simulink model "ProbeklausurLoesungR2021"  (R2021b)
settings: Solver=ode1  StartTime=0.0  StopTime=20  FixedStep=0.00001  RelTol=1e-3
values from neighbouring files (symbols this model uses):
  m = 4    [integrieren.m]
undefined symbols (not defined in the file or in its folder): C2
settings Model: Creator=PM  LastModifiedBy=metzler
settings SolverCC: AlgebraicLoopSolver=TrustRegion
settings DebuggingCC: AlgebraicLoopMsg=none  UnconnectedInputMsg=none  UnconnectedOutputMsg=none  UnconnectedLineMsg=none
settings ModelReferenceCC: EnableRefExpFcnMdlSchedulingChecks=off

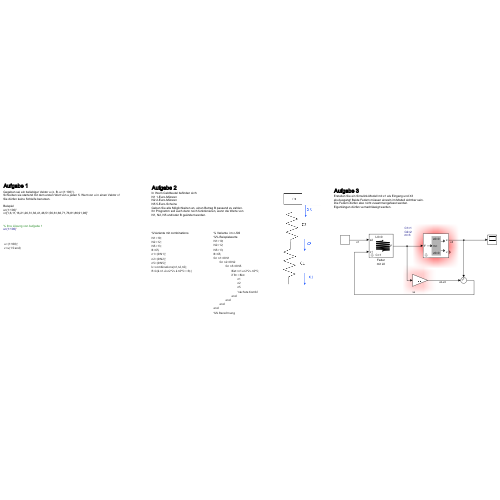
[thumbnail: Simulink's stored preview of the top-level diagram]
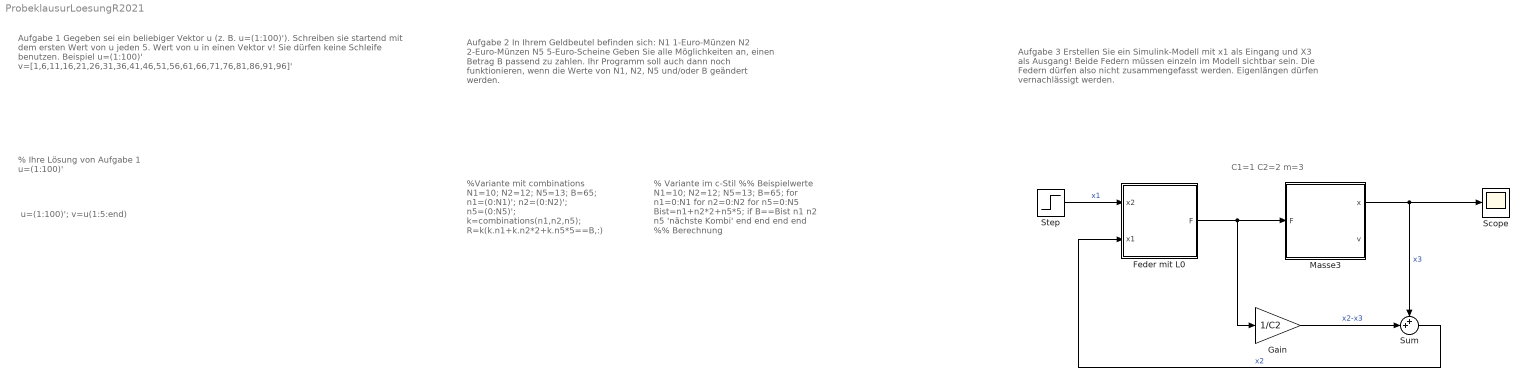
== system ProbeklausurLoesungR2021 ==
  note: Aufgabe 2
      | In Ihrem Geldbeutel befinden sich:
      | N1 1-Euro-Münzen
      | N2 2-Euro-Münzen
      | N5 5-Euro-Scheine
      | Geben Sie alle Möglichkeiten an, einen Betrag B passend zu zahlen.
      | Ihr Programm soll auch dann noch funktionieren, wenn die Werte von
      | N1, N2, N5 und/oder B geändert werden.
  note: Aufgabe 1
      | Gegeben sei ein beliebiger Vektor u (z. B. u=(1:100)').
      | Schreiben sie startend mit dem ersten Wert von u jeden 5. Wert von u in einen Vektor v!
      | Sie dürfen keine Schleife benutzen.
      |
      | Beispiel
      | u=(1:100)'
      | v=[1,6,11,16,21,26,31,36,41,46,51,56,61,66,71,76,81,86,91,96]'
  note: % Ihre Lösung von Aufgabe 1
      | u=(1:100)'
  note: Aufgabe 3
      | Erstellen Sie ein Simulink-Modell mit x1 als Eingang und X3
      | als Ausgang! Beide Federn müssen einzeln im Modell sichtbar sein.
      | Die Federn dürfen also nicht zusammengefasst werden.
      | Eigenlängen dürfen vernachlässigt werden.
  note: u=(1:100)';
      | v=u(1:5:end)
  note: %Variante mit combinations
      | N1=10;
      | N2=12;
      | N5=13;
      | B=65;
      | n1=(0:N1)';
      | n2=(0:N2)';
      | n5=(0:N5)';
      | k=combinations(n1,n2,n5);
      | R=k(k.n1+k.n2*2+k.n5*5==B,:)
  note: % Variante im c-Stil
      | %% Beispielwerte
      | N1=10;
      | N2=12;
      | N5=13;
      | B=65;
      | for n1=0:N1
      | for n2=0:N2
      | for n5=0:N5
      | Bist=n1+n2*2+n5*5;
      | if B==Bist
      | n1
      | n2
      | n5
      | 'nächste Kombi'
      | end
      | end
      | end
      | end
      | %% Berechnung
  note: C1=1
      | C2=2
      | m=3
  " Feder mit L0" : Subsystem  mask{C=1, L0=0}
      mask prompts: C "Spring Constant C [N/m]"; L0 "Length of Spring if no force is applied L0 [m]"
      mask help:
      | If no force F is applied, the spring has the length L0.
      |
      | F=C*sign(x2-x1-L0)*((x2-x1-L0)
      mask Display:
      | plot(20,0)
      | plot(90,100)
      | plot([60,60],[25,30])
      | plot([60,80],[30,32])
      | plot([80,40],[32,36])
      | plot([40,80],[36,40])
      | plot([80,40],[40,44])
      | plot([40,80],[44,48])
      | plot([80,40],[48,52])
      | plot([40,80],[52,56])
      | plot([80,40],[56,60])
      | plot([40,80],[60,64])
      | plot([80,40],[64,68])
      | plot([40,60],[68,70])
      | plot([60,60],[70,75])
      | 
      | 
      | port_label ('output',1,'F')
      | port_label ('input',1,'x2')
      | port_label ('input',2,'x1')
      | 
      | text(40,10,['C=',num2str(C)])
      | text(40,90,['L0=',num2str(L0)])
  Gain : Gain  Gain=1/C2
  Masse3 : Subsystem  mask{m=m, v0=0, x0=0}
      mask prompts: m "Masse m"; v0 "Anfangsgeschwindigkeit v_0"; x0 "Anfangsposition x_0"
      mask help:
      | Calculates the position s and the velocity v of a mass as a function of the Force F and the initial velocity v_0 and initial position s_0.
      | Berechnet die Position und die Geschwindigkeit eines Köpers mit der Masse m. Auf den Köper wirkt die Kraft F. Die Anfangsposition ist s_0, die Anfangsgeschwindigkeit ist v_0.
      mask Display:
      | plot(0,0)
      | plot(100,100)
      | patch([35 35 70 70],[10 90 90 10],[0.7,0.7,0.7])
      | text(40,80,['x0=',num2str(x0)])
      | text(40,50,['m=',num2str(m)])
      | text(40,20,['v0=',num2str(v0)])
      | plot([70 80],[70 70])
      | patch([80 80 85],[65 75 70],[0 0 0])
      | plot([15 35],[50 50])
      | patch([30 30 35],[45 55 50],[0 0 0])
      | plot([70 80],[30 30])
      | patch([80 80 85],[25 35 30],[0 0 0])
      | port_label ('output',1,'x')
      | port_label ('output',2,'v')
      | port_label ('input',1,'F')
  Scope : Scope
  Step : Step  SampleTime=0
  Sum : Sum  Inputs=++|
  wires:
  Sum/1 -> " Feder mit L0"/2(x1)  "x2"
  " Feder mit L0"/1(F) -> Gain/1, Masse3/1(F)
  Step/1 -> " Feder mit L0"/1(x2)  "x1"
  Gain/1 -> Sum/2  "x2-x3"
  Masse3/1(x) -> Scope/1, Sum/1  "x3"

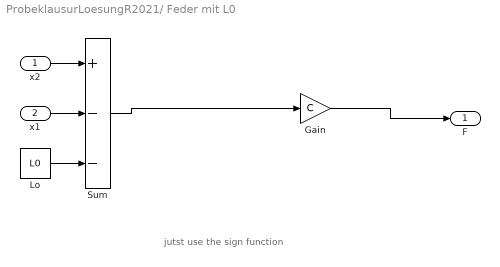
== system ProbeklausurLoesungR2021/ Feder mit L0 ==
  note: jutst use the sign function
  x2 : Inport
  x1 : Inport  Port=2
  Gain : Gain  Gain=C
  Lo : Constant  Value=L0
  Sum : Sum  Inputs=+--
  F : Outport  VectorParamsAs1DForOutWhenUnconnected=off
  wires:
  x2/1 -> Sum/1
  x1/1 -> Sum/2
  Lo/1 -> Sum/3
  Sum/1 -> Gain/1
  Gain/1 -> F/1

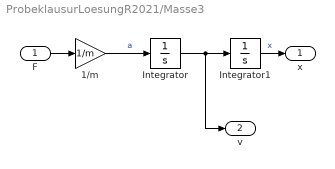
== system ProbeklausurLoesungR2021/Masse3 ==
  F : Inport
  1/m : Gain  Gain=1/m
  Integrator : Integrator  InitialCondition=v0
  Integrator1 : Integrator  InitialCondition=x0
  x : Outport  VectorParamsAs1DForOutWhenUnconnected=off
  v : Outport  Port=2  VectorParamsAs1DForOutWhenUnconnected=off
  wires:
  1/m/1 -> Integrator/1  "a"
  Integrator/1 -> Integrator1/1, v/1
  F/1 -> 1/m/1
  Integrator1/1 -> x/1  "x"
